simulink library "TripedLibrary"  (R2021a)
settings: Solver=VariableStepAuto  StartTime=0.0  StopTime=10.0  RelTol=1e-3
values from neighbouring files (symbols this model uses):
  s = 1/(2*r)    [Weg0.m]
undefined symbols (not defined in the file or in its folder): X, Y, Z
libraries: sm_lib x95, nesl_utility x42, $bdroot x14, robotlib x9, simulink x6, spsFirstOrderFilterLib x3, mspsensorlib x1
(part 1 of 5)
Description:
  | A library containing parts of the TriPed of the ARIES LAB at the Ziti at the University of Heidelberg.
settings Model: Creator=max  LastModifiedBy=jan-b
settings SolverCC: AlgebraicLoopSolver=TrustRegion
settings DebuggingCC: SFMachineParentedDataDiag=warning

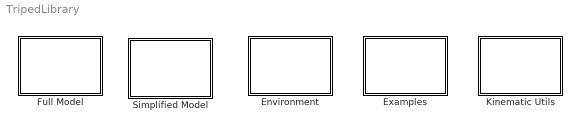
== system TripedLibrary ==
  Environment : Subsystem
  Examples : Subsystem
  Full Model : Subsystem
  Kinematic Utils : Subsystem
  Simplified Model : Subsystem

== system TripedLibrary/Environment ==
  Grounds : Subsystem
  World to Robot Switch : Subsystem  Variant=on  VariantControlMode=label  LabelModeActiveChoice=Choice_2

== system TripedLibrary/Examples ==
  Full Body orientation and height control : Subsystem
  Initialisation : Subsystem
  Rotating Chassis : Subsystem
  Spider Walking : Subsystem
  Swinging Chassis : Subsystem
  rabbid walking : Subsystem

== system TripedLibrary/Full Model ==
  Parts : Subsystem
  ROS : Subsystem
  TriPed : Subsystem
      mask Display: image('./icons/full_triped_logo.png')

== system TripedLibrary/Kinematic Utils ==
  Full Model kinematics : Subsystem
  Simplified  Model Kinematics : Subsystem
  fullbody kinematics : MATLAB Function  TreatAsAtomicUnit=on

== system TripedLibrary/Simplified Model ==
  Parts : Subsystem
  ROS : Subsystem
  TriPed : Subsystem
      settings: PortSchema="{\"entries\":[{\"content\":{\"sides\":[{\"content\":{\"connectorIds\":[\"In1\",\"LConn1\"]},\"type\":\"ConnectorPlacement.EquallySpacedRectSide\",\"uuid\":\"cf937cc4-9946-458f-a00c-c6b64d50e5dd\"},{\"content\":{\"connectorIds\":[\"RConn1\",\"RConn2\",\"RConn3\",\"Out1\"],\"side\":\"RIGHT\"},\"type\":\"ConnectorPlacement.EquallySpacedRectSide\",\"uuid\":\"24e17f8e-a145-44bf-b20e-4a80bbb5751f\"},{\"content\":{\"connectorIds\":[],\"side\":\"TOP\"},\"type\":\"ConnectorPlacement.EquallySpacedRectSide\",\"uuid\":\"6e43fe6c-017a-4e02-a518-41141b50f8f7\"}]},\"type\":\"ConnectorPlacement.EquallySpacedConnector\",\"uuid\":\"8dc904d1-a5ef-4597-b7a1-5eba3e01f89e\"}],\"packageUris\":[\"http://schema.mathworks.com/mf0/Connector/19700101\"],\"version\":\"1.0\"}"
      mask Display: image('./icons/simplified_triped_logo.png')

== system TripedLibrary/Environment/Grounds ==
  Ground_Rubber_on_Concrete : Subsystem

== system TripedLibrary/Environment/World to Robot Switch ==
  note: 1) Add Subsystem or Model blocks as valid variant choices.
      | 2) You cannot connect blocks at this level. At simulation, connectivity is automatically
      | determined, based on the active variant and port name matching.
  Free : Subsystem  VariantControl=Choice_2
  Rigid : Subsystem  VariantControl=(default)
  World frame : PMIOPort  Side=Left
  Connection Port1 : PMIOPort  Port=2  Side=Right

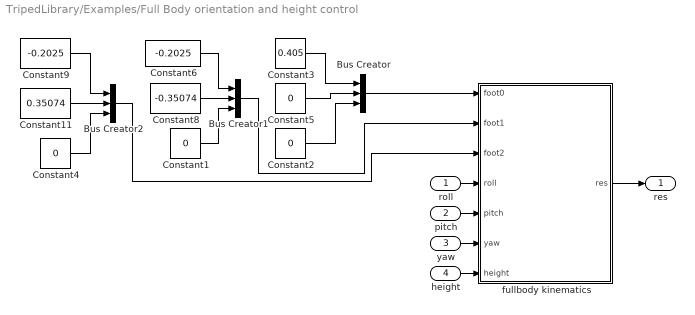
== system TripedLibrary/Examples/Full Body orientation and height control ==
  roll : Inport
  pitch : Inport  Port=2
  yaw : Inport  Port=3
  height : Inport  Port=4
  Bus Creator : BusCreator  Inputs=3
  Bus Creator1 : BusCreator  Inputs=3
  Bus Creator2 : BusCreator  Inputs=3
  Constant{1..2,4..5} (4 alike) : Constant  Value=0
  Constant11 : Constant  Value=0.35074
  Constant3 : Constant  Value=0.405
  Constant6 : Constant  Value=-0.2025
  Constant8 : Constant  Value=-0.35074
  Constant9 : Constant  Value=-0.2025
  fullbody kinematics : MATLAB Function  TreatAsAtomicUnit=on
  res : Outport
  wires:
  Bus Creator2/1 -> fullbody kinematics/3(foot2)
  pitch/1 -> fullbody kinematics/5(pitch)
  roll/1 -> fullbody kinematics/4(roll)
  height/1 -> fullbody kinematics/7(height)
  fullbody kinematics/1(res) -> res/1
  Bus Creator/1 -> fullbody kinematics/1(foot0)
  Bus Creator1/1 -> fullbody kinematics/2(foot1)
  yaw/1 -> fullbody kinematics/6(yaw)
  Constant5/1 -> Bus Creator/2
  Constant3/1 -> Bus Creator/1
  Constant2/1 -> Bus Creator/3
  Constant8/1 -> Bus Creator1/2
  Constant6/1 -> Bus Creator1/1
  Constant1/1 -> Bus Creator1/3
  Constant11/1 -> Bus Creator2/2
  Constant9/1 -> Bus Creator2/1
  Constant4/1 -> Bus Creator2/3

== system TripedLibrary/Examples/Initialisation ==
  note: Initialisation
  note: Initialiszes the system to a height of 60 cm above ground
  Bus Creator1 : BusCreator  Inputs=9
  Constant11 : Constant  Value=0.35074
  Constant3 : Constant  Value=0.405
  Constant5 : Constant  Value=0
  Constant6 : Constant  Value=-0.2025
  Constant8 : Constant  Value=-0.35074
  Constant9 : Constant  Value=-0.2025
  Ramp : simulink/Sources/Ramp  slope=-0.3  start=0  InitialOutput=-0.023  VectorParams1D=off
  Saturation : Saturate  LowerLimit=-0.6
  Out1 : Outport
  wires:
  Constant9/1 -> Bus Creator1/7
  Constant5/1 -> Bus Creator1/2
  Constant6/1 -> Bus Creator1/4
  Constant3/1 -> Bus Creator1/1
  Saturation/1 -> Bus Creator1/3, Bus Creator1/6, Bus Creator1/9
  Constant8/1 -> Bus Creator1/5
  Constant11/1 -> Bus Creator1/8
  Bus Creator1/1 -> Out1/1
  Ramp/1 -> Saturation/1

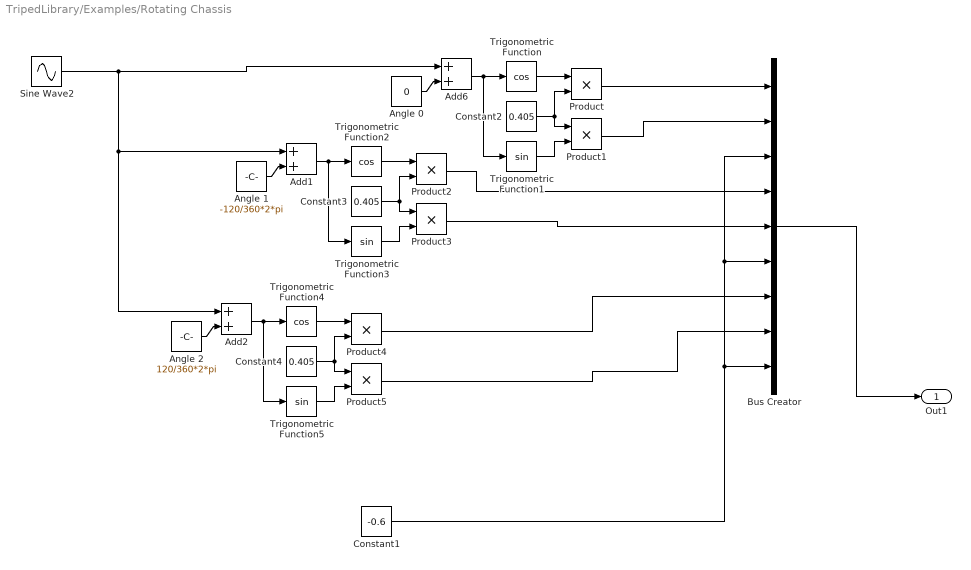
== system TripedLibrary/Examples/Rotating Chassis ==
  Add1 : Sum
  Add2 : Sum
  Add6 : Sum
  Angle 0 : Constant  Value=0
  Angle 1 : Constant  Value=-120/360*2*pi
  Angle 2 : Constant  Value=120/360*2*pi
  Bus Creator : BusCreator  Inputs=9
  Constant1 : Constant  Value=-0.6
  Constant2 : Constant  Value=0.405
  Constant3 : Constant  Value=0.405
  Constant4 : Constant  Value=0.405
  Product{,1..5} (6 alike) : Product
  Sine Wave2 : Sin  Frequency=pi  SampleTime=0
  Trigonometric Function : Trigonometry  Operator=cos
  Trigonometric Function1 : Trigonometry
  Trigonometric Function2 : Trigonometry  Operator=cos
  Trigonometric Function3 : Trigonometry
  Trigonometric Function4 : Trigonometry  Operator=cos
  Trigonometric Function5 : Trigonometry
  Out1 : Outport
  wires:
  Constant1/1 -> Bus Creator/3, Bus Creator/6, Bus Creator/9
  Bus Creator/1 -> Out1/1
  Angle 0/1 -> Add6/2
  Add6/1 -> Trigonometric Function1/1, Trigonometric Function/1
  Trigonometric Function/1 -> Product/1
  Constant2/1 -> Product/2, Product1/1
  Trigonometric Function1/1 -> Product1/2
  Product/1 -> Bus Creator/1
  Product1/1 -> Bus Creator/2
  Constant3/1 -> Product2/2, Product3/1
  Trigonometric Function3/1 -> Product3/2
  Trigonometric Function2/1 -> Product2/1
  Angle 1/1 -> Add1/2
  Add1/1 -> Trigonometric Function3/1, Trigonometric Function2/1
  Product2/1 -> Bus Creator/4
  Product3/1 -> Bus Creator/5
  Add2/1 -> Trigonometric Function5/1, Trigonometric Function4/1
  Angle 2/1 -> Add2/2
  Sine Wave2/1 -> Add2/1, Add1/1, Add6/1
  Trigonometric Function5/1 -> Product5/2
  Trigonometric Function4/1 -> Product4/1
  Constant4/1 -> Product4/2, Product5/1
  Product4/1 -> Bus Creator/7
  Product5/1 -> Bus Creator/8

== system TripedLibrary/Examples/Spider Walking ==
  note: Choose Walking Angle
      | relative to X Axis
  Bus Creator1 : BusCreator  Inputs=3
  Gait Generator : MATLAB Function  TreatAsAtomicUnit=on  SystemSampleTime=0.01
  Knob : KnobBlock  ScaleMax=360
  Unit Delay1 : UnitDelay  InitialCondition=[0 0 0 0 0 0 0 0 0]  SampleTime=-1  HasFrameUpgradeWarning=on
  Unit Delay2 : UnitDelay  InitialCondition=3*pi  SampleTime=-1  HasFrameUpgradeWarning=on
  Walking dir : Constant  Value=0
  Out1 : Outport
  wires:
  Bus Creator1/1 -> Out1/1, Unit Delay1/1
  Gait Generator/1(foot_0) -> Bus Creator1/1
  Gait Generator/2(foot_1) -> Bus Creator1/2
  Gait Generator/3(foot_2) -> Bus Creator1/3
  Unit Delay1/1 -> Gait Generator/1(current_foot_pos)
  Gait Generator/4(angle) -> Unit Delay2/1
  Unit Delay2/1 -> Gait Generator/2("angle ")
  Walking dir/1 -> Gait Generator/3(walking_dir)

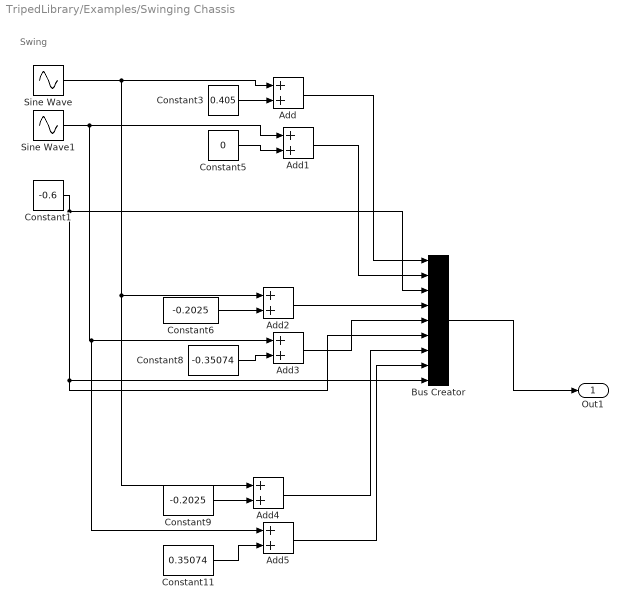
== system TripedLibrary/Examples/Swinging Chassis ==
  note: Swing
  Add{,1..5} (6 alike) : Sum
  Bus Creator : BusCreator  Inputs=9
  Constant1 : Constant  Value=-0.6
  Constant11 : Constant  Value=0.35074
  Constant3 : Constant  Value=0.405
  Constant5 : Constant  Value=0
  Constant6 : Constant  Value=-0.2025
  Constant8 : Constant  Value=-0.35074
  Constant9 : Constant  Value=-0.2025
  Sine Wave : Sin  Amplitude=0.1  Frequency=pi  SampleTime=0
  Sine Wave1 : Sin  Amplitude=0.1  Frequency=pi  Phase=pi/2  SampleTime=0
  Out1 : Outport
  wires:
  Add1/1 -> Bus Creator/2
  Add4/1 -> Bus Creator/7
  Add3/1 -> Bus Creator/5
  Constant1/1 -> Bus Creator/3, Bus Creator/6, Bus Creator/9
  Add/1 -> Bus Creator/1
  Add5/1 -> Bus Creator/8
  Add2/1 -> Bus Creator/4
  Bus Creator/1 -> Out1/1
  Constant6/1 -> Add2/2
  Constant8/1 -> Add3/2
  Constant9/1 -> Add4/2
  Constant5/1 -> Add1/2
  Sine Wave/1 -> Add4/1, Add2/1, Add/1
  Constant11/1 -> Add5/2
  Constant3/1 -> Add/2
  Sine Wave1/1 -> Add5/1, Add3/1, Add1/1

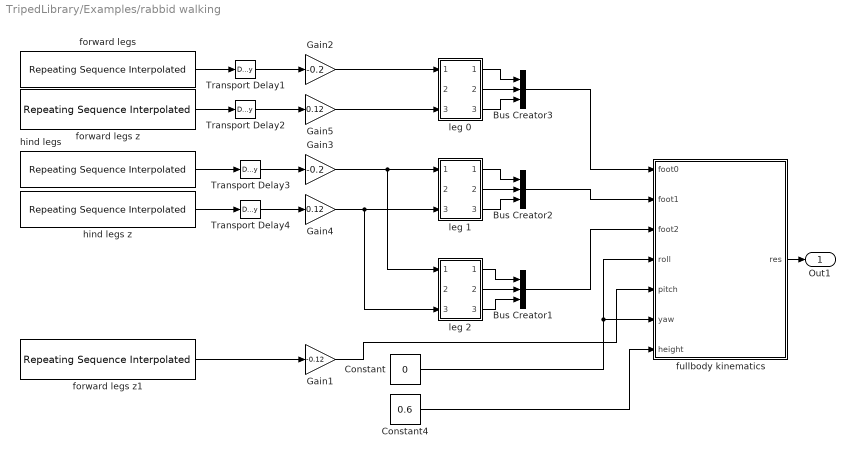
== system TripedLibrary/Examples/rabbid walking ==
  Bus Creator1 : BusCreator  Inputs=3
  Bus Creator2 : BusCreator  Inputs=3
  Bus Creator3 : BusCreator  Inputs=3
  Constant : Constant  Value=0
  Constant4 : Constant  Value=0.6
  Gain1 : Gain  Gain=-0.12
  Gain2 : Gain  Gain=-0.2
  Gain3 : Gain  Gain=-0.2
  Gain4 : Gain  Gain=0.12
  Gain5 : Gain  Gain=0.12
  Transport Delay{1..4} (4 alike) : TransportDelay  DelayTime=0.2
  forward legs : simulink/Sources/Repeating Sequence Interpolated  OutValues="[0 1 1  -1 0].'"  TimeValues=[0 0.25 0.9 1 1.2 ].'  LookUpMeth=Interpolation-Use End Values  tsamp=0.01  OutMin=[]  OutMax=[]  OutDataTypeStr=double  OutputDataTypeScalingMode=double  OutDataType=fixdt(0,8)  OutScaling=2^-10
  forward legs z : simulink/Sources/Repeating Sequence Interpolated  OutValues="[0 0 0 1  0 00].'"  TimeValues="[0 0.25  0.9 0.91  1.15  1.2 ].'"  LookUpMeth=Interpolation-Use End Values  tsamp=0.01  OutMin=[]  OutMax=[]  OutDataTypeStr=double  OutputDataTypeScalingMode=double  OutDataType=fixdt(0,8)  OutScaling=2^-10
  forward legs z1 : simulink/Sources/Repeating Sequence Interpolated  OutValues="[0 0 1 1  0 00].'"  TimeValues="[0 0.25  0.9 0.91  1.15  1.2 ].'"  LookUpMeth=Interpolation-Use End Values  tsamp=0.01  OutMin=[]  OutMax=[]  OutDataTypeStr=double  OutputDataTypeScalingMode=double  OutDataType=fixdt(0,8)  OutScaling=2^-10
  fullbody kinematics : MATLAB Function  TreatAsAtomicUnit=on
  hind legs : simulink/Sources/Repeating Sequence Interpolated  OutValues="[0 1 0  0 0 ].'"  TimeValues="[0 0.25  0.8 0.95 1.2].'"  LookUpMeth=Interpolation-Use End Values  tsamp=0.01  OutMin=[]  OutMax=[]  OutDataTypeStr=double  OutputDataTypeScalingMode=double  OutDataType=fixdt(0,8)  OutScaling=2^-10
  hind legs z : simulink/Sources/Repeating Sequence Interpolated  OutValues="[0 0 1 1 0  0 ].'"  TimeValues="[0 0.25  0.26 0.525 0.8  1.2 ].'"  LookUpMeth=Interpolation-Use End Values  tsamp=0.01  OutMin=[]  OutMax=[]  OutDataTypeStr=double  OutputDataTypeScalingMode=double  OutDataType=fixdt(0,8)  OutScaling=2^-10
  leg 0 : Subsystem
  leg 1 : Subsystem
  leg 2 : Subsystem
  Out1 : Outport
  wires:
  leg 0/1(Out1) -> Bus Creator3/1
  leg 0/2(Out2) -> Bus Creator3/2
  leg 0/3(Out3) -> Bus Creator3/3
  leg 1/1(Out1) -> Bus Creator2/1
  leg 1/2(Out2) -> Bus Creator2/2
  leg 1/3(Out3) -> Bus Creator2/3
  leg 2/1(Out1) -> Bus Creator1/1
  leg 2/2(Out2) -> Bus Creator1/2
  leg 2/3(Out3) -> Bus Creator1/3
  Gain4/1 -> leg 2/3(In3), leg 1/3(In3)
  Gain2/1 -> leg 0/1(In1)
  forward legs/1 -> Transport Delay1/1
  hind legs/1 -> Transport Delay3/1
  Gain3/1 -> leg 2/1(In1), leg 1/1(In1)
  hind legs z/1 -> Transport Delay4/1
  forward legs z/1 -> Transport Delay2/1
  Gain5/1 -> leg 0/3(In3)
  Transport Delay1/1 -> Gain2/1
  Transport Delay2/1 -> Gain5/1
  Transport Delay3/1 -> Gain3/1
  Transport Delay4/1 -> Gain4/1
  fullbody kinematics/1(res) -> Out1/1
  Bus Creator3/1 -> fullbody kinematics/1(foot0)
  Bus Creator2/1 -> fullbody kinematics/2(foot1)
  Bus Creator1/1 -> fullbody kinematics/3(foot2)
  Constant/1 -> fullbody kinematics/6(yaw), fullbody kinematics/4(roll)
  Constant4/1 -> fullbody kinematics/7(height)
  Gain1/1 -> fullbody kinematics/5(pitch)
  forward legs z1/1 -> Gain1/1

== system TripedLibrary/Full Model/Parts ==
  AS5047D Hall Sensor : Subsystem
      mask Display: image('./icons/hall_sensor.png'); % Use "Edit Image" on toolstrip to change.
  Chassis : $bdroot/Full Model/TriPed/Chassis  SystemSampleTime=-1  VariantActivationTime=update diagram  Latency=0  AutoFrameSizeCalculation=off
  E6A2-C Rotary Encoder : Subsystem
      mask Display: image('./icons/incremental_sensor.png'); % Use "Edit Image" on toolstrip to change.
  Leg : Subsystem
      mask Display:
      | image('./icons/triped_leg_kinematic_new_colors.png')
      | port_label('input',1,'MotorSignals')
      | port_label('output',1,'SensorSignals')
      | port_label('rconn',1,'GroundConnection')

== system TripedLibrary/Full Model/ROS ==
  Publisher_leg_0 : Subsystem
  Subscriber_leg0 : Subsystem

== system TripedLibrary/Full Model/TriPed ==
  Joint_commands : Inport
  Chassis : Subsystem
  Demux : Demux  Outputs=3
  Leg : $bdroot/Full Model/Parts/Leg  SystemSampleTime=-1  VariantActivationTime=update diagram  Latency=0  AutoFrameSizeCalculation=off
  Leg1 : $bdroot/Full Model/Parts/Leg  SystemSampleTime=-1  VariantActivationTime=update diagram  Latency=0  AutoFrameSizeCalculation=off
  Leg2 : $bdroot/Full Model/Parts/Leg  SystemSampleTime=-1  VariantActivationTime=update diagram  Latency=0  AutoFrameSizeCalculation=off
  Mux : Mux  Inputs=3
  Rotate_Leg : sm_lib/Frames and Transforms/Rigid Transform  TranslationMethod=None  TranslationStandardOffset=0  TranslationLengthUnit=m  TranslationStandardAxis=+Z  TranslationCartesianOffset=[0 0 0]  TranslationROffset=0  TranslationROffsetUnits=m  TranslationZOffset=0  TranslationZOffsetUnits=m  TranslationThetaOffset=0  TranslationThetaOffsetUnits=deg  RotationMethod=StandardAxis  RotationAngleUnits=deg  RotationStandardAxis=+Z  RotationAngle=0 * -120  RotationArbitraryAxis=[0 0 1]  FollAlignAxisA=+X  BaseAlignAxisA=+Y  FollAlignAxisB=+Y  BaseAlignAxisB=+Z  RotationSequenceAxes=FollowerAxes  RotationSequence=XYX  RotationSequenceAngles=[0 0 0]  RotationSequenceAnglesUnits=deg  RotationMatrix=[1 0 0; 0 1 0; 0 0 1]
  Rotate_Leg1 : sm_lib/Frames and Transforms/Rigid Transform  TranslationMethod=None  TranslationStandardOffset=0  TranslationLengthUnit=m  TranslationStandardAxis=+Z  TranslationCartesianOffset=[0 0 0]  TranslationROffset=0  TranslationROffsetUnits=m  TranslationZOffset=0  TranslationZOffsetUnits=m  TranslationThetaOffset=0  TranslationThetaOffsetUnits=deg  RotationMethod=StandardAxis  RotationAngleUnits=deg  RotationStandardAxis=+Z  RotationAngle=1 * -120  RotationArbitraryAxis=[0 0 1]  FollAlignAxisA=+X  BaseAlignAxisA=+Y  FollAlignAxisB=+Y  BaseAlignAxisB=+Z  RotationSequenceAxes=FollowerAxes  RotationSequence=XYX  RotationSequenceAngles=[0 0 0]  RotationSequenceAnglesUnits=deg  RotationMatrix=[1 0 0; 0 1 0; 0 0 1]
  Rotate_Leg2 : sm_lib/Frames and Transforms/Rigid Transform  TranslationMethod=None  TranslationStandardOffset=0  TranslationLengthUnit=m  TranslationStandardAxis=+Z  TranslationCartesianOffset=[0 0 0]  TranslationROffset=0  TranslationROffsetUnits=m  TranslationZOffset=0  TranslationZOffsetUnits=m  TranslationThetaOffset=0  TranslationThetaOffsetUnits=deg  RotationMethod=StandardAxis  RotationAngleUnits=deg  RotationStandardAxis=+Z  RotationAngle=2 * -120  RotationArbitraryAxis=[0 0 1]  FollAlignAxisA=+X  BaseAlignAxisA=+Y  FollAlignAxisB=+Y  BaseAlignAxisB=+Z  RotationSequenceAxes=FollowerAxes  RotationSequence=XYX  RotationSequenceAngles=[0 0 0]  RotationSequenceAnglesUnits=deg  RotationMatrix=[1 0 0; 0 1 0; 0 0 1]
  World_to_Robot_Connection : PMIOPort  Side=Left
  leg0_Ground_Connection : PMIOPort  Port=2  Side=Right
  leg1_Ground_Connection : PMIOPort  Port=3  Side=Right
  leg2_Ground_Connection : PMIOPort  Port=4  Side=Right
  Sensors : Outport
  wires:
  Demux/2 -> Leg1/1
  Demux/3 -> Leg/1
  Leg2/1 -> Mux/1
  Leg1/1 -> Mux/2
  Leg/1 -> Mux/3
  Demux/1 -> Leg2/1
  Mux/1 -> Sensors/1
  Joint_commands/1 -> Demux/1
  connections:
  Rotate_Leg2/LConn1 -- Rotate_Leg1/LConn1 -- Rotate_Leg/LConn1 -- Chassis/LConn1 -- World_to_Robot_Connection/RConn1
  leg0_Ground_Connection/RConn1 -- Leg2/LConn2
  leg1_Ground_Connection/RConn1 -- Leg1/LConn2
  leg2_Ground_Connection/RConn1 -- Leg/LConn2
  Rotate_Leg2/RConn1 -- Leg/LConn1
  Leg1/LConn1 -- Rotate_Leg1/RConn1
  Leg2/LConn1 -- Rotate_Leg/RConn1

== system TripedLibrary/Kinematic Utils/Full Model kinematics ==

== system TripedLibrary/Kinematic Utils/Simplified  Model Kinematics ==
  Fwd Kin : MATLAB Function  TreatAsAtomicUnit=on
  Inv Kin : Subsystem

== system TripedLibrary/Simplified Model/Parts ==
  Chassis : $bdroot/Simplified Model/TriPed/Chassis  SystemSampleTime=-1  VariantActivationTime=update diagram  Latency=0  AutoFrameSizeCalculation=off
  Simplified Leg : Subsystem
      mask Display: image('./icons/triped_leg_kinematic_new_colors.png')

== system TripedLibrary/Simplified Model/ROS ==
  note: TODO

== system TripedLibrary/Simplified Model/TriPed ==
  note: Click on the small gray arrow to view the Leg Subsystem
  desired_foot_position : Inport
  Chassis : Subsystem
  Forward Kinematics : Subsystem
      settings: PortSchema="{\"entries\":[{\"content\":{\"sides\":[{\"content\":{\"connectorIds\":[\"Out1\"]},\"type\":\"ConnectorPlacement.EquallySpacedRectSide\",\"uuid\":\"723aa903-851a-4664-882b-cb687275721b\"},{\"content\":{\"connectorIds\":[\"RConn1\",\"In1\",\"In2\",\"In3\"],\"side\":\"RIGHT\"},\"type\":\"ConnectorPlacement.EquallySpacedRectSide\",\"uuid\":\"f9e95ccf-8a42-4456-81db-8f425e241ec1\"},{\"content\":{\"connectorIds\":[],\"side\":\"TOP\"},\"type\":\"ConnectorPlacement.EquallySpacedRectSide\",\"uuid\":\"175b5798-3047-4472-9bca-bb6c2911fede\"}]},\"type\":\"ConnectorPlacement.EquallySpacedConnector\",\"uuid\":\"62df2873-5e03-4e99-98e6-e4829089aed6\"}],\"packageUris\":[\"http://schema.mathworks.com/mf0/Connector/19700101\"],\"version\":\"1.0\"}"
  Inverse Kinematics : Subsystem
      settings: PortSchema="{\"entries\":[{\"content\":{\"sides\":[{\"content\":{\"connectorIds\":[\"In1\"]},\"type\":\"ConnectorPlacement.EquallySpacedRectSide\",\"uuid\":\"cacf1049-8908-4031-8a69-d560fb3daf87\"},{\"content\":{\"connectorIds\":[\"Out1\",\"Out2\",\"Out3\"],\"side\":\"RIGHT\"},\"type\":\"ConnectorPlacement.EquallySpacedRectSide\",\"uuid\":\"44d3a5e5-b5a5-4353-9f1f-1978183a0ef7\"},{\"content\":{\"connectorIds\":[\"LConn1\"],\"side\":\"TOP\"},\"type\":\"ConnectorPlacement.EquallySpacedRectSide\",\"uuid\":\"35953bc0-548a-45fe-829f-cc09c83310c3\"}]},\"type\":\"ConnectorPlacement.EquallySpacedConnector\",\"uuid\":\"2cbed19f-c886-4304-b559-6e30441489df\"}],\"packageUris\":[\"http://schema.mathworks.com/mf0/Connector/19700101\"],\"version\":\"1.0\"}"
  Rotate_Leg : sm_lib/Frames and Transforms/Rigid Transform  TranslationMethod=None  TranslationStandardOffset=0  TranslationLengthUnit=m  TranslationStandardAxis=+Z  TranslationCartesianOffset=[0 0 0]  TranslationROffset=0  TranslationROffsetUnits=m  TranslationZOffset=0  TranslationZOffsetUnits=m  TranslationThetaOffset=0  TranslationThetaOffsetUnits=deg  RotationMethod=StandardAxis  RotationAngleUnits=deg  RotationStandardAxis=+Z  RotationAngle=0 * -120  RotationArbitraryAxis=[0 0 1]  FollAlignAxisA=+X  BaseAlignAxisA=+Y  FollAlignAxisB=+Y  BaseAlignAxisB=+Z  RotationSequenceAxes=FollowerAxes  RotationSequence=XYX  RotationSequenceAngles=[0 0 0]  RotationSequenceAnglesUnits=deg  RotationMatrix=[1 0 0; 0 1 0; 0 0 1]
  Rotate_Leg1 : sm_lib/Frames and Transforms/Rigid Transform  TranslationMethod=None  TranslationStandardOffset=0  TranslationLengthUnit=m  TranslationStandardAxis=+Z  TranslationCartesianOffset=[0 0 0]  TranslationROffset=0  TranslationROffsetUnits=m  TranslationZOffset=0  TranslationZOffsetUnits=m  TranslationThetaOffset=0  TranslationThetaOffsetUnits=deg  RotationMethod=StandardAxis  RotationAngleUnits=deg  RotationStandardAxis=+Z  RotationAngle=1 * -120  RotationArbitraryAxis=[0 0 1]  FollAlignAxisA=+X  BaseAlignAxisA=+Y  FollAlignAxisB=+Y  BaseAlignAxisB=+Z  RotationSequenceAxes=FollowerAxes  RotationSequence=XYX  RotationSequenceAngles=[0 0 0]  RotationSequenceAnglesUnits=deg  RotationMatrix=[1 0 0; 0 1 0; 0 0 1]
  Rotate_Leg2 : sm_lib/Frames and Transforms/Rigid Transform  TranslationMethod=None  TranslationStandardOffset=0  TranslationLengthUnit=m  TranslationStandardAxis=+Z  TranslationCartesianOffset=[0 0 0]  TranslationROffset=0  TranslationROffsetUnits=m  TranslationZOffset=0  TranslationZOffsetUnits=m  TranslationThetaOffset=0  TranslationThetaOffsetUnits=deg  RotationMethod=StandardAxis  RotationAngleUnits=deg  RotationStandardAxis=+Z  RotationAngle=2 * -120  RotationArbitraryAxis=[0 0 1]  FollAlignAxisA=+X  BaseAlignAxisA=+Y  FollAlignAxisB=+Y  BaseAlignAxisB=+Z  RotationSequenceAxes=FollowerAxes  RotationSequence=XYX  RotationSequenceAngles=[0 0 0]  RotationSequenceAnglesUnits=deg  RotationMatrix=[1 0 0; 0 1 0; 0 0 1]
  Simplified Leg : $bdroot/Simplified Model/Parts/Simplified Leg  SystemSampleTime=-1  VariantActivationTime=update diagram  Latency=0  AutoFrameSizeCalculation=off
  Simplified Leg1 : $bdroot/Simplified Model/Parts/Simplified Leg  SystemSampleTime=-1  VariantActivationTime=update diagram  Latency=0  AutoFrameSizeCalculation=off
  Simplified Leg2 : $bdroot/Simplified Model/Parts/Simplified Leg  SystemSampleTime=-1  VariantActivationTime=update diagram  Latency=0  AutoFrameSizeCalculation=off
  World_to_Robot_Connection : PMIOPort  Side=Left
  leg0_Ground_Connection : PMIOPort  Port=2  Side=Right
  leg1_Ground_Connection : PMIOPort  Port=3  Side=Right
  leg2_Ground_Connection1 : PMIOPort  Port=4  Side=Right
  current_foot_position : Outport
  wires:
  Inverse Kinematics/2(Leg1Bus) -> Simplified Leg1/1
  Inverse Kinematics/3(Leg2Bus) -> Simplified Leg2/1
  desired_foot_position/1 -> Inverse Kinematics/1(In1)
  Simplified Leg/1 -> Forward Kinematics/1(Leg0Bus)
  Simplified Leg1/1 -> Forward Kinematics/2(Leg1Bus)
  Simplified Leg2/1 -> Forward Kinematics/3(Leg2Bus)
  Forward Kinematics/1(foot positions) -> current_foot_position/1
  Inverse Kinematics/1(Leg0Bus) -> Simplified Leg/1
  connections:
  Simplified Leg/LConn2 -- leg0_Ground_Connection/RConn1
  Simplified Leg1/LConn2 -- leg1_Ground_Connection/RConn1
  Simplified Leg2/LConn2 -- leg2_Ground_Connection1/RConn1
  Rotate_Leg1/LConn1 -- Rotate_Leg2/LConn1 -- Rotate_Leg/LConn1 -- World_to_Robot_Connection/RConn1 -- Inverse Kinematics/LConn1 -- Chassis/LConn1
  Chassis/RConn1 -- Forward Kinematics/RConn1
  Simplified Leg/LConn1 -- Rotate_Leg/RConn1
  Simplified Leg1/LConn1 -- Rotate_Leg1/RConn1
  Rotate_Leg2/RConn1 -- Simplified Leg2/LConn1

== system TripedLibrary/Environment/Grounds/Ground_Rubber_on_Concrete ==
  note: Setup Ground
  note: Compute Robot-Ground Force
  note: Quantise_Leg_Forces
  First-Order Filter : spsFirstOrderFilterLib/First-Order Filter  FilterType=Lowpass  Tc=1/30  Ts=0  Initialize=on  Vac_Init=[0, 0, 60]  Vdc_Init=0  PlotResponse=off  FreqRange="[0,  200,  1]"
  First-Order Filter1 : spsFirstOrderFilterLib/First-Order Filter  FilterType=Lowpass  Tc=1/30  Ts=0  Initialize=on  Vac_Init=[0, 0, 60]  Vdc_Init=0  PlotResponse=off  FreqRange="[0,  200,  1]"
  First-Order Filter2 : spsFirstOrderFilterLib/First-Order Filter  FilterType=Lowpass  Tc=1/30  Ts=0  Initialize=on  Vac_Init=[0, 0, 60]  Vdc_Init=0  PlotResponse=off  FreqRange="[0,  200,  1]"
  Ground : sm_lib/Body Elements/Brick Solid  GraphicAmbientColor=[0.15 0.15 0.15 1.0]  BasedOnType=Density  BrickDimensions=[4 4 0.1]  BrickDimensionUnits=m  CenterOfMass=[0 0 0]  CenterOfMassUnits=m  GraphicDiffuseColor=[0.4 0.4 0.4]  Density=1000  DensityUnits=kg/m^3  DoExposeReferenceFrame=on  GraphicEmissiveColor=[0.0 0.0 0.0 1.0]  ExportEntireGeometry=on  SerializedFrames=<Frames/>  MarkerShape=Sphere  MarkerSize=10  GraphicType=FromGeometry  InertiaType=CalculateFromGeometry  Mass=1  MassUnits=kg  MomentsOfInertia=[1 1 1]  MomentsOfInertiaUnits=kg*m^2  GraphicOpacity=0.8  ProductsOfInertia=[0 0 0]  ProductsOfInertiaUnits=kg*m^2  GraphicShininess=75  GraphicSpecularColor=[0.5 0.5 0.5 1.0]  GraphicVisPropType=SimpleVisualProperties
  Ground_Connection : sm_lib/Joints/Weld Joint  JointMode=Normal  SenseConstraintForce=off  SenseConstraintForceX=off  SenseConstraintForceY=off  SenseConstraintForceZ=off  SenseConstraintTorque=off  SenseConstraintTorqueX=off  SenseConstraintTorqueY=off  SenseConstraintTorqueZ=off  SenseTotalForce=off  SenseTotalForceX=off  SenseTotalForceY=off  SenseTotalForceZ=off  SenseTotalTorque=off  SenseTotalTorqueX=off  SenseTotalTorqueY=off  SenseTotalTorqueZ=off  CompositeWrenchDir=FollowerOnBase  CompositeWrenchFrame=BaseFrame
  PS-Simulink Converter : nesl_utility/PS-Simulink Converter  PhysicalDomain=network_engine_domain  SubClassName=ps_output  LeftPortType=input  RightPortType=output  PseudoPeriodic=off  Frequencies=[]  Unit=inherit  AffineConversion=off
      settings: SourceProductBaseCode=PW,SS
  PS-Simulink Converter1 : nesl_utility/PS-Simulink Converter  PhysicalDomain=network_engine_domain  SubClassName=ps_output  LeftPortType=input  RightPortType=output  PseudoPeriodic=off  Frequencies=[]  Unit=inherit  AffineConversion=off
      settings: SourceProductBaseCode=PW,SS
  PS-Simulink Converter2 : nesl_utility/PS-Simulink Converter  PhysicalDomain=network_engine_domain  SubClassName=ps_output  LeftPortType=input  RightPortType=output  PseudoPeriodic=off  Frequencies=[]  Unit=inherit  AffineConversion=off
      settings: SourceProductBaseCode=PW,SS
  SpatialContactForce-Leg0 : sm_lib/Forces and Torques/Spatial Contact Force  CoefficientOfDynamicFriction=0.3  CoefficientOfStaticFriction=1  SenseContactBaseRotation=off  SenseContactBaseTranslation=off  NormalDamping=1e4  NormalDampingUnits=N/(m/s)  SenseContactFollowerRotation=off  SenseContactFollowerTranslation=off  SenseContactSignal=off  NormalStiffness=1e6  NormalStiffnessUnits=N/m  FrictionalCriticalVelocity=1e-3  FrictionalCriticalVelocityUnits=m/s  ZeroCrossDetectContactStartAndEnd=on  FrictionType=SmoothStickSlip  SenseFrictionalForceMagnitude=off  SenseNormalForceMagnitude=on  NormalForceType=SmoothSpringDamper  SenseNormalVelocity=off  SenseSeparationDistance=off  SenseTangentialVelocity=off  SenseTangentialVelocityMagnitude=off  NormalTransitionRegionWidth=1e-4  NormalTransitionRegionWidthUnits=m
  SpatialContactForce-Leg1 : sm_lib/Forces and Torques/Spatial Contact Force  CoefficientOfDynamicFriction=0.3  CoefficientOfStaticFriction=1  SenseContactBaseRotation=off  SenseContactBaseTranslation=off  NormalDamping=1e4  NormalDampingUnits=N/(m/s)  SenseContactFollowerRotation=off  SenseContactFollowerTranslation=off  SenseContactSignal=off  NormalStiffness=1e6  NormalStiffnessUnits=N/m  FrictionalCriticalVelocity=1e-3  FrictionalCriticalVelocityUnits=m/s  ZeroCrossDetectContactStartAndEnd=on  FrictionType=SmoothStickSlip  SenseFrictionalForceMagnitude=off  SenseNormalForceMagnitude=on  NormalForceType=SmoothSpringDamper  SenseNormalVelocity=off  SenseSeparationDistance=off  SenseTangentialVelocity=off  SenseTangentialVelocityMagnitude=off  NormalTransitionRegionWidth=1e-4  NormalTransitionRegionWidthUnits=m
  SpatialContactForce-Leg2 : sm_lib/Forces and Torques/Spatial Contact Force  CoefficientOfDynamicFriction=0.3  CoefficientOfStaticFriction=1  SenseContactBaseRotation=off  SenseContactBaseTranslation=off  NormalDamping=1e4  NormalDampingUnits=N/(m/s)  SenseContactFollowerRotation=off  SenseContactFollowerTranslation=off  SenseContactSignal=off  NormalStiffness=1e6  NormalStiffnessUnits=N/m  FrictionalCriticalVelocity=1e-3  FrictionalCriticalVelocityUnits=m/s  ZeroCrossDetectContactStartAndEnd=on  FrictionType=SmoothStickSlip  SenseFrictionalForceMagnitude=off  SenseNormalForceMagnitude=on  NormalForceType=SmoothSpringDamper  SenseNormalVelocity=off  SenseSeparationDistance=off  SenseTangentialVelocity=off  SenseTangentialVelocityMagnitude=off  NormalTransitionRegionWidth=1e-4  NormalTransitionRegionWidthUnits=m
  World_to_Ground : PMIOPort  Side=Left
  Force_GND_to_Leg_2 : PMIOPort  Port=2  Side=Right
  Force_GND_to_Leg_1 : PMIOPort  Port=3  Side=Right
  Force_GND_to_Leg_0 : PMIOPort  Port=4  Side=Right
  wires:
  PS-Simulink Converter2/1 -> First-Order Filter2/1
  PS-Simulink Converter1/1 -> First-Order Filter1/1
  PS-Simulink Converter/1 -> First-Order Filter/1
  First-Order Filter/1 -> ?
  First-Order Filter1/1 -> ?
  First-Order Filter2/1 -> ?
  connections:
  Ground/RConn1 -- Ground_Connection/RConn1
  Ground/LConn1 -- SpatialContactForce-Leg0/LConn1 -- SpatialContactForce-Leg1/LConn1 -- SpatialContactForce-Leg2/LConn1
  SpatialContactForce-Leg1/RConn1 -- Force_GND_to_Leg_1/RConn1
  SpatialContactForce-Leg2/RConn1 -- Force_GND_to_Leg_2/RConn1
  SpatialContactForce-Leg0/RConn1 -- Force_GND_to_Leg_0/RConn1
  World_to_Ground/RConn1 -- Ground_Connection/LConn1
  PS-Simulink Converter1/LConn1 -- SpatialContactForce-Leg1/RConn2
  PS-Simulink Converter2/LConn1 -- SpatialContactForce-Leg2/RConn2
  PS-Simulink Converter/LConn1 -- SpatialContactForce-Leg0/RConn2

== system TripedLibrary/Environment/World to Robot Switch/Free ==
  World_to_CCS_6-DOF-Joint : sm_lib/Joints/6-DOF Joint  JointMode=Normal  SenseConstraintForce=off  SenseConstraintForceX=off  SenseConstraintForceY=off  SenseConstraintForceZ=off  SenseConstraintTorque=off  SenseConstraintTorqueX=off  SenseConstraintTorqueY=off  SenseConstraintTorqueZ=off  SenseTotalForce=off  SenseTotalForceX=off  SenseTotalForceY=off  SenseTotalForceZ=off  SenseTotalTorque=off  SenseTotalTorqueX=off  SenseTotalTorqueY=off  SenseTotalTorqueZ=off  CompositeWrenchDir=FollowerOnBase  CompositeWrenchFrame=BaseFrame  PxEquilibriumPosition=0  PxEquilibriumPositionUnits=m  PxSpringStiffness=0  PxSpringStiffnessUnits=N/m  PxDampingCoefficient=0  PxDampingCoefficientUnits=N/(m/s)  PxTorqueActuationMode=NoTorque  PxMotionActuationMode=ComputedMotion  PxSensePosition=off  PxSenseVelocity=off  PxSenseAcceleration=off  PxSenseTorqueForce=off  PxSenseLowerLimitTorqueForce=off  PxSenseUpperLimitTorqueForce=off  PxLowerLimitSpecify=off  PxLowerLimitBound=-1  PxLowerLimitBoundUnits=m  PxLowerLimitStiffness=1e6  PxLowerLimitStiffnessUnits=N/m  PxLowerLimitDamping=1e3  PxLowerLimitDampingUnits=N/(m/s)  PxLowerLimitTransitionRegionWidth=1e-4  PxLowerLimitTransitionRegionWidthUnits=m  PxUpperLimitSpecify=off  PxUpperLimitBound=1  PxUpperLimitBoundUnits=m  PxUpperLimitStiffness=1e6  PxUpperLimitStiffnessUnits=N/m  PxUpperLimitDamping=1e3  PxUpperLimitDampingUnits=N/(m/s)  PxUpperLimitTransitionRegionWidth=1e-4  PxUpperLimitTransitionRegionWidthUnits=m  PxPositionTargetSpecify=off  PxPositionTargetPriority=High  PxPositionTargetValue=0  PxPositionTargetValueUnits=m  PxVelocityTargetSpecify=off  PxVelocityTargetPriority=High  PxVelocityTargetValue=0  PxVelocityTargetValueUnits=m/s  PyEquilibriumPosition=0  PyEquilibriumPositionUnits=m  PySpringStiffness=0  PySpringStiffnessUnits=N/m  PyDampingCoefficient=0  PyDampingCoefficientUnits=N/(m/s)  PyTorqueActuationMode=NoTorque  PyMotionActuationMode=ComputedMotion  PySensePosition=off  PySenseVelocity=off  PySenseAcceleration=off  PySenseTorqueForce=off  PySenseLowerLimitTorqueForce=off  PySenseUpperLimitTorqueForce=off  PyLowerLimitSpecify=off  PyLowerLimitBound=-1  PyLowerLimitBoundUnits=m  PyLowerLimitStiffness=1e6  PyLowerLimitStiffnessUnits=N/m  PyLowerLimitDamping=1e3  PyLowerLimitDampingUnits=N/(m/s)  PyLowerLimitTransitionRegionWidth=1e-4  PyLowerLimitTransitionRegionWidthUnits=m  PyUpperLimitSpecify=off  PyUpperLimitBound=1  PyUpperLimitBoundUnits=m  PyUpperLimitStiffness=1e6  PyUpperLimitStiffnessUnits=N/m  PyUpperLimitDamping=1e3  PyUpperLimitDampingUnits=N/(m/s)  PyUpperLimitTransitionRegionWidth=1e-4  PyUpperLimitTransitionRegionWidthUnits=m  PyPositionTargetSpecify=off  PyPositionTargetPriority=High  PyPositionTargetValue=0  PyPositionTargetValueUnits=m  PyVelocityTargetSpecify=off  PyVelocityTargetPriority=High  PyVelocityTargetValue=0  PyVelocityTargetValueUnits=m/s  PzEquilibriumPosition=0  PzEquilibriumPositionUnits=m  PzSpringStiffness=0  PzSpringStiffnessUnits=N/m  PzDampingCoefficient=0  PzDampingCoefficientUnits=N/(m/s)  PzTorqueActuationMode=NoTorque  PzMotionActuationMode=ComputedMotion  PzSensePosition=off  PzSenseVelocity=off  PzSenseAcceleration=off  PzSenseTorqueForce=off  PzSenseLowerLimitTorqueForce=off  PzSenseUpperLimitTorqueForce=off  PzLowerLimitSpecify=off  PzLowerLimitBound=-1  PzLowerLimitBoundUnits=m  PzLowerLimitStiffness=1e6  PzLowerLimitStiffnessUnits=N/m  PzLowerLimitDamping=1e3  PzLowerLimitDampingUnits=N/(m/s)  PzLowerLimitTransitionRegionWidth=1e-4  PzLowerLimitTransitionRegionWidthUnits=m  PzUpperLimitSpecify=off  PzUpperLimitBound=1  PzUpperLimitBoundUnits=m  PzUpperLimitStiffness=1e6  PzUpperLimitStiffnessUnits=N/m  PzUpperLimitDamping=1e3  PzUpperLimitDampingUnits=N/(m/s)  PzUpperLimitTransitionRegionWidth=1e-4  PzUpperLimitTransitionRegionWidthUnits=m  PzPositionTargetSpecify=off  PzPositionTargetPriority=High  PzPositionTargetValue=0  PzPositionTargetValueUnits=m  PzVelocityTargetSpecify=off  PzVelocityTargetPriority=High  PzVelocityTargetValue=0  PzVelocityTargetValueUnits=m/s  SphDefPosRotationMethod=None  SphDefPosRotationAngleUnits=deg  SphDefPosRotationStandardAxis=+Z  SphDefPosRotationAngle=0.0  SphDefPosRotationArbitraryAxis=[0 0 1]  SphDefPosFollAlignAxisA=+X  SphDefPosBaseAlignAxisA=+Y  SphDefPosFollAlignAxisB=+Y  SphDefPosBaseAlignAxisB=+Z  SphDefPosRotationSequenceAxes=FollowerAxes  SphDefPosRotationSequence=XYX  SphDefPosRotationSequenceAngles=[0 0 0]  SphDefPosRotationSequenceAnglesUnits=deg  SphDefPosRotationMatrix=[1 0 0; 0 1 0; 0 0 1]  SphEqPosRotationMethod=None  SphEqPosRotationAngleUnits=deg  SphEqPosRotationStandardAxis=+Z  SphEqPosRotationAngle=0.0  SphEqPosRotationArbitraryAxis=[0 0 1]  SphEqPosFollAlignAxisA=+X  SphEqPosBaseAlignAxisA=+Y  SphEqPosFollAlignAxisB=+Y  SphEqPosBaseAlignAxisB=+Z  SphEqPosRotationSequenceAxes=FollowerAxes  SphEqPosRotationSequence=XYX  SphEqPosRotationSequenceAngles=[0 0 0]  SphEqPosRotationSequenceAnglesUnits=deg  SphEqPosRotationMatrix=[1 0 0; 0 1 0; 0 0 1]  SphSpringStiffness=0  SphSpringStiffnessUnits=N*m/deg  SphDampingCoefficient=0  SphDampingCoefficientUnits=N*m/(deg/s)  SphActuateTorqueX=off  SphActuateTorqueY=off  SphActuateTorqueZ=off  SphActuateTorque=off  SphTorqueActuationMode=NoTorque  SphMotionActuationMode=ComputedMotion  SphActuationFrame=BaseFrame  SphSensePosition=off  SphSenseVelocityX=off  SphSenseVelocityY=off  SphSenseVelocityZ=off  SphSenseVelocity=off  SphSenseAccelerationX=off  SphSenseAccelerationY=off  SphSenseAccelerationZ=off  SphSenseAcceleration=off  SphSenseTorqueX=off  SphSenseTorqueY=off  SphSenseTorqueZ=off  SphSenseTorqueForce=off  SphSenseLowerLimitTorqueMag=off  SphSenseUpperLimitTorqueMag=off  SphSensingFrame=BaseFrame  SphLowerLimitSpecify=off  SphLowerLimitBound=15  SphLowerLimitBoundUnits=deg  SphLowerLimitStiffness=1e4  SphLowerLimitStiffnessUnits=N*m/deg  SphLowerLimitDamping=10  SphLowerLimitDampingUnits=N*m/(deg/s)  SphLowerLimitTransitionRegionWidth=0.1  SphLowerLimitTransitionRegionWidthUnits=deg  SphUpperLimitSpecify=off  SphUpperLimitBound=45  SphUpperLimitBoundUnits=deg  SphUpperLimitStiffness=1e4  SphUpperLimitStiffnessUnits=N*m/deg  SphUpperLimitDamping=10  SphUpperLimitDampingUnits=N*m/(deg/s)  SphUpperLimitTransitionRegionWidth=0.1  SphUpperLimitTransitionRegionWidthUnits=deg  SphPositionTargetRotationMethod=None  SphPositionTargetRotationAngleUnits=deg  SphPositionTargetRotationStandardAxis=+Z  SphPositionTargetRotationAngle=0.0  SphPositionTargetRotationArbitraryAxis=[0 0 1]  SphPositionTargetFollAlignAxisA=+X  SphPositionTargetBaseAlignAxisA=+Y  SphPositionTargetFollAlignAxisB=+Y  SphPositionTargetBaseAlignAxisB=+Z  SphPositionTargetRotationSequenceAxes=FollowerAxes  SphPositionTargetRotationSequence=XYX  SphPositionTargetRotationSequenceAngles=[0 0 0]  SphPositionTargetRotationSequenceAnglesUnits=deg  SphPositionTargetRotationMatrix=[1 0 0; 0 1 0; 0 0 1]  SphPositionTargetSpecify=off  SphPositionTargetPriority=High  SphVelocityTargetValue=[0 0 0]  SphVelocityTargetValueUnits=deg/s  SphVelocityTargetSpecify=off  SphVelocityTargetPriority=High  SphVelocityTargetInFollowerFrame=on
  World frame : PMIOPort  Side=Left
  Connection Port1 : PMIOPort  Port=2  Side=Right
  connections:
  World_to_CCS_6-DOF-Joint/RConn1 -- Connection Port1/RConn1
  World_to_CCS_6-DOF-Joint/LConn1 -- World frame/RConn1

== system TripedLibrary/Environment/World to Robot Switch/Rigid ==
  World_to_CCS : sm_lib/Joints/Weld Joint  JointMode=Normal  SenseConstraintForce=off  SenseConstraintForceX=off  SenseConstraintForceY=off  SenseConstraintForceZ=off  SenseConstraintTorque=off  SenseConstraintTorqueX=off  SenseConstraintTorqueY=off  SenseConstraintTorqueZ=off  SenseTotalForce=off  SenseTotalForceX=off  SenseTotalForceY=off  SenseTotalForceZ=off  SenseTotalTorque=off  SenseTotalTorqueX=off  SenseTotalTorqueY=off  SenseTotalTorqueZ=off  CompositeWrenchDir=FollowerOnBase  CompositeWrenchFrame=BaseFrame
  World frame : PMIOPort  Side=Left
  Connection Port1 : PMIOPort  Port=2  Side=Right
  connections:
  World_to_CCS/RConn1 -- Connection Port1/RConn1
  World frame/RConn1 -- World_to_CCS/LConn1

== system TripedLibrary/Examples/rabbid walking/leg 0 ==
  In1 : Inport
  In2 : Inport  Port=2
  In3 : Inport  Port=3
  Add : Sum
  Add1 : Sum
  Add10 : Sum
  Constant10 : Constant  Value=0
  Constant3 : Constant  Value=0.405
  Constant5 : Constant  Value=0
  Out1 : Outport
  Out2 : Outport  Port=2
  Out3 : Outport  Port=3
  wires:
  Add1/1 -> Out2/1
  Constant5/1 -> Add1/2
  Constant10/1 -> Add10/2
  Add10/1 -> Out3/1
  In2/1 -> Add1/1
  Constant3/1 -> Add/2
  Add/1 -> Out1/1
  In3/1 -> Add10/1
  In1/1 -> Add/1

== system TripedLibrary/Examples/rabbid walking/leg 1 ==
  In1 : Inport
  In2 : Inport  Port=2
  In3 : Inport  Port=3
  Add2 : Sum
  Add3 : Sum
  Add9 : Sum
  Constant6 : Constant  Value=-0.2025
  Constant7 : Constant  Value=0
  Constant8 : Constant  Value=-0.35074
  Gain : Gain  Gain=1.3
  Gain1 : Gain  Gain=1.3
  Out1 : Outport
  Out2 : Outport  Port=2
  Out3 : Outport  Port=3
  wires:
  In3/1 -> Add9/1
  Constant6/1 -> Gain/1
  Add9/1 -> Out3/1
  Add2/1 -> Out1/1
  Constant8/1 -> Gain1/1
  Constant7/1 -> Add9/2
  Add3/1 -> Out2/1
  In2/1 -> Add3/1
  In1/1 -> Add2/1
  Gain/1 -> Add2/2
  Gain1/1 -> Add3/2

== system TripedLibrary/Examples/rabbid walking/leg 2 ==
  In1 : Inport
  In2 : Inport  Port=2
  In3 : Inport  Port=3
  Add4 : Sum
  Add5 : Sum
  Add8 : Sum
  Constant11 : Constant  Value=0.35074
  Constant4 : Constant  Value=0
  Constant9 : Constant  Value=-0.2025
  Gain : Gain  Gain=1.3
  Gain1 : Gain  Gain=1.3
  Out1 : Outport
  Out2 : Outport  Port=2
  Out3 : Outport  Port=3
  wires:
  In2/1 -> Add5/1
  Constant11/1 -> Gain/1
  In3/1 -> Add8/1
  Constant9/1 -> Gain1/1
  Add5/1 -> Out2/1
  Add8/1 -> Out3/1
  Constant4/1 -> Add8/2
  Add4/1 -> Out1/1
  In1/1 -> Add4/1
  Gain1/1 -> Add4/2
  Gain/1 -> Add5/2

== system TripedLibrary/Full Model/Parts/AS5047D Hall Sensor ==
  In2 : Inport
  Add1 : Sum
  Quantizer : Quantizer  QuantizationInterval=2*pi/2048
  Random Number1 : RandomNumber  Mean=1  Variance=0.002^2 /3  SampleTime=0
  Out2 : Outport
  wires:
  Random Number1/1 -> Add1/2
  Add1/1 -> Quantizer/1
  In2/1 -> Add1/1
  Quantizer/1 -> Out2/1

== system TripedLibrary/Full Model/Parts/E6A2-C Rotary Encoder ==
  In1 : Inport
  Add : Sum
  Quantizer2 : Quantizer  QuantizationInterval=2*pi/500
  Random Number : RandomNumber  Variance=0.002^2 /3  SampleTime=0
  Out1 : Outport
  wires:
  Quantizer2/1 -> Out1/1
  In1/1 -> Add/1
  Add/1 -> Quantizer2/1
  Random Number/1 -> Add/2

== system TripedLibrary/Full Model/Parts/Leg ==
  joint_commands : Inport
  Demux : Demux  Outputs=3
  Gear conversion : Gain  Gain=(2*pi*1.5)/0.07
  Mux : Mux  Inputs=3
  OpenSubChain : Subsystem
      settings: PortSchema="{\"entries\":[{\"content\":{\"sides\":[{\"content\":{\"connectorIds\":[\"In1\",\"LConn1\"]},\"type\":\"ConnectorPlacement.EquallySpacedRectSide\",\"uuid\":\"19c1487c-dda0-4172-8025-939be1e4895f\"},{\"content\":{\"connectorIds\":[\"Out1\",\"RConn1\"],\"side\":\"RIGHT\"},\"type\":\"ConnectorPlacement.EquallySpacedRectSide\",\"uuid\":\"1d2fa5a6-f45f-4ff4-b41b-f562edb1766a\"},{\"content\":{\"connectorIds\":[],\"side\":\"TOP\"},\"type\":\"ConnectorPlacement.EquallySpacedRectSide\",\"uuid\":\"081b96ad-1671-4e19-8a74-8977369d5a36\"},{\"content\":{\"connectorIds\":[\"RConn2\"],\"side\":\"BOTTOM\"},\"type\":\"ConnectorPlacement.EquallySpacedRectSide\",\"uuid\":\"7d233002-b0fd-449b-8dc6-383b89e193f4\"}]},\"type\":\"ConnectorPlacement.EquallySpacedConnector\",\"uuid\":\"a40c46d9-0848-4a96-9047-bae3eb8225dd\"}],\"packageUris\":[\"http://schema.mathworks.com/mf0/Connector/19700101\"],\"version\":\"1.0\"}"
      mask Display: image('./icons/open_chain.png'); % Use "Edit Image" on toolstrip to change.
  Sensor Modelling : Subsystem
      settings: PortSchema="{\"entries\":[{\"content\":{\"sides\":[{\"content\":{\"connectorIds\":[\"LConn1\",\"In1\",\"LConn2\",\"LConn3\"]},\"type\":\"ConnectorPlacement.EquallySpacedRectSide\",\"uuid\":\"8c1b8b91-02bd-491b-8ffe-53b2b5a44dfb\"},{\"content\":{\"connectorIds\":[\"Out1\",\"Out2\",\"Out3\"],\"side\":\"RIGHT\"},\"type\":\"ConnectorPlacement.EquallySpacedRectSide\",\"uuid\":\"b3a0e2d1-c457-44ea-850c-fac9c104df03\"},{\"content\":{\"connectorIds\":[],\"side\":\"TOP\"},\"type\":\"ConnectorPlacement.EquallySpacedRectSide\",\"uuid\":\"c6cd551a-4849-410a-8d21-185d6b3380c4\"}]},\"type\":\"ConnectorPlacement.EquallySpacedConnector\",\"uuid\":\"44729963-7c66-43d7-89da-497d266c8e29\"}],\"packageUris\":[\"http://schema.mathworks.com/mf0/Connector/R2020b\"],\"version\":\"1.0\"}"
  SubChain 0 : Subsystem
      mask Display: image('./icons/chain_0.png'); % Use "Edit Image" on toolstrip to change.
  SubChain 1 : Subsystem
      mask Display: image('./icons/chain_1.png'); % Use "Edit Image" on toolstrip to change.
  SubChain 2 : Subsystem
      mask Display: image('./icons/chain_2.png'); % Use "Edit Image" on toolstrip to change.
  Leg_CCS_Connection : PMIOPort  Side=Left
  Leg_to_Ground_Force_Connection : PMIOPort  Port=2  Side=Left
  joint_states : Outport
  wires:
  OpenSubChain/1(Accelerometer_Out) -> Sensor Modelling/1(accelerometer)
  Demux/3 -> SubChain 1/1(input0)
  Demux/1 -> SubChain 2/1(input0)
  Sensor Modelling/1(srs_quant) -> Mux/1
  Demux/2 -> Gear conversion/1
  Sensor Modelling/2(ses_quant) -> Mux/2
  joint_commands/1 -> Demux/1
  Sensor Modelling/3(sls_quant) -> Mux/3
  Mux/1 -> joint_states/1
  Gear conversion/1 -> OpenSubChain/1(input0)
  connections:
  OpenSubChain/LConn1 -- SubChain 1/RConn1 -- SubChain 2/RConn2 -- SubChain 0/RConn1
  SubChain 0/LConn1 -- Leg_CCS_Connection/RConn1 -- SubChain 1/LConn1 -- SubChain 2/LConn1
  OpenSubChain/RConn1 -- Sensor Modelling/LConn2
  Sensor Modelling/LConn3 -- SubChain 1/RConn2
  SubChain 2/RConn1 -- Sensor Modelling/LConn1
  Leg_to_Ground_Force_Connection/RConn1 -- OpenSubChain/RConn2

== system TripedLibrary/Full Model/ROS/Publisher_leg_0 ==
  In Bus Element : Inport  PortName=motor_quantized_position  Element=swing_left_motor_quantized_position
  In Bus Element1 : Inport  PortName=motor_quantized_position  Element=swing_right_motor_quantized_position
  In Bus Element2 : Inport  PortName=motor_quantized_position  Element=extend_motor_quatized_position
  Sensor_Publisher : Subsystem  mask(Motor Publisher){topic=/leg0/swing/left/sensor}
      mask prompts: topic "ros:slros:blockmask:TopicPrompt"
      mask help: This is a sample description
      mask TypeOptions topic: RosPublisher/topic
      mask DialogControl topic Prompt: Topic:
      mask Display: block_icon('RosPublisher')
  Sensor_Publisher1 : Subsystem  mask(Motor Publisher){topic=/leg0/swing/right/sensor}
      mask prompts: topic "ros:slros:blockmask:TopicPrompt"
      mask help: This is a sample description
      mask TypeOptions topic: RosPublisher/topic
      mask DialogControl topic Prompt: Topic:
      mask Display: block_icon('RosPublisher')
  Sensor_Publisher2 : Subsystem  mask(Motor Publisher){topic=/leg0/extend/sensor}
      mask prompts: topic "ros:slros:blockmask:TopicPrompt"
      mask help: This is a sample description
      mask TypeOptions topic: RosPublisher/topic
      mask DialogControl topic Prompt: Topic:
      mask Display: block_icon('RosPublisher')
  wires:
  In Bus Element1/1 -> Sensor_Publisher1/1(position)
  In Bus Element2/1 -> Sensor_Publisher2/1(position)
  In Bus Element/1 -> Sensor_Publisher/1(position)

== system TripedLibrary/Full Model/ROS/Subscriber_leg0 ==
  Ros-Subscriber-leg-0-extend-motor : Subsystem
  Ros-Subscriber-leg-0-left-swing-motor : Subsystem
  Ros-Subscriber-leg-0-right-swing-motor : Subsystem
  Out Bus Element : Outport  PortName=Leg0Bus_OUT  Element=swing_left_motor.position
  Out Bus Element1 : Outport  PortName=Leg0Bus_OUT  Element=swing_left_motor.velocity
  Out Bus Element2 : Outport  PortName=Leg0Bus_OUT  Element=swing_left_motor.effort
  Out Bus Element3 : Outport  PortName=Leg0Bus_OUT  Element=swing_right_motor.position
  Out Bus Element4 : Outport  PortName=Leg0Bus_OUT  Element=swing_right_motor.velocity
  Out Bus Element5 : Outport  PortName=Leg0Bus_OUT  Element=swing_right_motor.effort
  Out Bus Element6 : Outport  PortName=Leg0Bus_OUT  Element=extend_motor.position
  Out Bus Element7 : Outport  PortName=Leg0Bus_OUT  Element=extend_motor.velocity
  Out Bus Element8 : Outport  PortName=Leg0Bus_OUT  Element=extend_motor.effort
  wires:
  Ros-Subscriber-leg-0-extend-motor/2(extend_motor_velocity_OUT) -> Out Bus Element7/1
  Ros-Subscriber-leg-0-right-swing-motor/2(swing_right_motor_velocity_OUT) -> Out Bus Element4/1
  Ros-Subscriber-leg-0-extend-motor/1(extend_motor_position_OUT) -> Out Bus Element6/1
  Ros-Subscriber-leg-0-extend-motor/3(extend_motor_effort_OUT) -> Out Bus Element8/1
  Ros-Subscriber-leg-0-left-swing-motor/2(swing_left_motor_velocity_OUT) -> Out Bus Element1/1
  Ros-Subscriber-leg-0-right-swing-motor/3(swing_right_motor_effort_OUT) -> Out Bus Element5/1
  Ros-Subscriber-leg-0-left-swing-motor/3(swing_left_motor_effort_OUT) -> Out Bus Element2/1
  Ros-Subscriber-leg-0-right-swing-motor/1(swing_right_motor_position_OUT) -> Out Bus Element3/1
  Ros-Subscriber-leg-0-left-swing-motor/1(swing_left_motor_position_OUT) -> Out Bus Element/1

== system TripedLibrary/Full Model/TriPed/Chassis ==
  Chassis : sm_lib/Body Elements/File Solid  ExtGeomFileName=./triped-files/CHASSIS_überarbeitet.stl  UnitType=Custom  ExtGeomFileUnits=mm  StepReaderType=HEX  ExportConvexHullGeometry=off  InertiaType=Custom  Mass=9.273  MassUnits=kg  CenterOfMass=[0 0 10.44]  CenterOfMassUnits=mm  MomentsOfInertia=[0.121 0.121 0.199]  MomentsOfInertiaUnits=kg*m^2  ProductsOfInertia=[0 0 0]  ProductsOfInertiaUnits=kg*m^2  BasedOnType=DensityFromFile  Density=1000  DensityUnits=kg/m^3  DoExposeReferenceFrame=on  SerializedFrames=<Frames/>  GraphicType=FromGeometry  MarkerShape=Sphere  MarkerSize=10  GraphicVisPropType=SimpleVisualProperties  GraphicDiffuseColor=[0.6 0.6 0.6]  GraphicSpecularColor=[0.5 0.5 0.5 1.0]  GraphicAmbientColor=[0.15 0.15 0.15 1.0]  GraphicEmissiveColor=[0.0 0.0 0.0 1.0]  GraphicShininess=75  GraphicOpacity=1
  visualize CCS : Subsystem
  " Chassis_connection" : PMIOPort  Side=Left
  connections:
  Chassis/RConn1 -- visualize CCS/LConn1 -- " Chassis_connection"/RConn1

== system TripedLibrary/Kinematic Utils/Simplified  Model Kinematics/Inv Kin ==
  x : Inport
  y : Inport  Port=2
  z : Inport  Port=3
  Leg Angle : Inport  Port=4
  Bus Creator : BusCreator  Inputs=4
  Simplified_inverse_kinematics : MATLAB Function  TreatAsAtomicUnit=on
  Transport Delay{,1..3} (4 alike) : TransportDelay  DelayTime=0.01
  Unit Delay : UnitDelay  InitialCondition=[0 0 0 0]  SampleTime=-1  HasFrameUpgradeWarning=on
  Out Bus Element : Outport  PortName=Leg0Bus_OUT  Element=gimbal_joint.Rx
  Out Bus Element1 : Outport  PortName=Leg0Bus_OUT  Element=gimbal_joint.Ry
  Out Bus Element2 : Outport  PortName=Leg0Bus_OUT  Element=gimbal_joint.Rz
  Out Bus Element6 : Outport  PortName=Leg0Bus_OUT  Element=extend_motor.position
  wires:
  Simplified_inverse_kinematics/5(Residual) -> ?
  Transport Delay/1 -> Out Bus Element6/1
  Bus Creator/1 -> Unit Delay/1
  y/1 -> Simplified_inverse_kinematics/2(y)
  Transport Delay2/1 -> Out Bus Element1/1
  Simplified_inverse_kinematics/3(Ry) -> Transport Delay2/1, Bus Creator/2
  Unit Delay/1 -> Simplified_inverse_kinematics/5(data)
  Transport Delay3/1 -> Out Bus Element2/1
  Leg Angle/1 -> Simplified_inverse_kinematics/4(LegAngle)
  x/1 -> Simplified_inverse_kinematics/1(x)
  z/1 -> Simplified_inverse_kinematics/3(z)
  Simplified_inverse_kinematics/1(extend) -> Transport Delay/1, Bus Creator/4
  Simplified_inverse_kinematics/4(Rz) -> Transport Delay3/1, Bus Creator/3
  Simplified_inverse_kinematics/2(Rx) -> Transport Delay1/1, Bus Creator/1
  Transport Delay1/1 -> Out Bus Element/1
